simulink model "Detumbling"  (R2023b)
settings: Solver=VariableStepAuto  StartTime=0.0  StopTime=10.0  RelTol=1e-3
values from neighbouring files (symbols this model uses):
  a = 7259    [Group_51.m]
  ARW = (((arw*pi/180)/(sqrt(n_t)))^2)*n_t    [Group_51.m]
  Beta_CMG = acos(dot([1;0;0],uv_pyr))    [Group_51.m]
  delta_0_D = zeros(4,1)    [Group_51.m]
  e = 0.001    [Group_51.m]
  eps_b = 11.5*pi/180    (= 0.200712863979)    [Group_51.m]
  f0 = deg2rad(0)    [Group_51.m]
  g_1_0 = -29404.8    [Group_51.m]
  g_1_1 = -1450.9    [Group_51.m]
  Gain_G = eye(3,3)    [Group_51.m]
  h_1_1 = 4653.5    [Group_51.m]
  h_r = [0.5;0.5;0.5;0.5]    [Group_51.m]
  halfrange = pi/40    (= 0.0785398163397)    [Group_51.m]
  i = deg2rad(97.27276)    [Group_51.m]
  I = diag(I)    [Group_51.m]
  I_inv = I\eye(3,3)    [Group_51.m]
  IC312_D = [phi312_D;theta312_D;psi312_D]    [Group_51.m]
  jb = [0.1; 0.1;0.1]    [Group_51.m]
  k_cmg = -1    [Group_51.m]
  kdx_D = 0.9896    [Group_51.m]
  kdy_D = 0.9734    [Group_51.m]
  kdz_D = 0.9096    [Group_51.m]
  Miss_G = [teta_g_x;teta_g_y;teta_g_z]    [Group_51.m]
  n = sqrt(mu/ a^3)    [Group_51.m]
  n_t = samp_t    (= 1)    [Group_51.m]
  OM = deg2rad(90)    [Group_51.m]
  Re = astroConstants(23)    [Group_51.m]
  RRW = (((rrw*pi/180)/(sqrt(n_t)))^2)*n_t    [Group_51.m]
  samp_t = 1/samp_freq    (= 1)    [Group_51.m]
  w = deg2rad(0)    [Group_51.m]
  w0_D = [wx_D;wy_D;wz_D]    [Group_51.m]
  w_t_D = zeros(3,1)    [Group_51.m]
  we = we/3600    (= 7.29159776389e-06)    [Group_51.m]
undefined symbols (not defined in the file or in its folder): DiscIntNeverNeededParam
libraries: matrix_library x7, vrlib x4, simulink x2, hdlsllib x2, dspswit3 x1
(part 1 of 2)
settings Model: Creator=leo-deo  LastModifiedBy=leo-deo

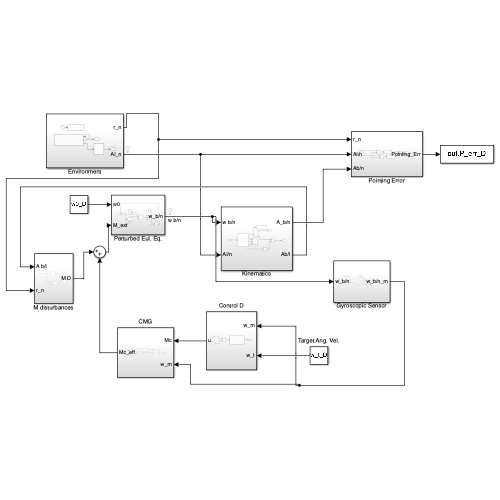
[thumbnail: Simulink's stored preview of the top-level diagram]
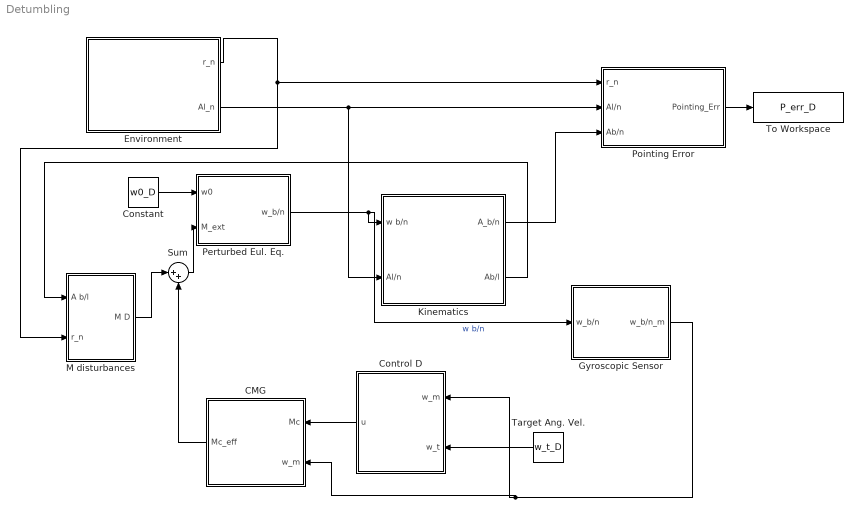
== system Detumbling ==
  CMG : Subsystem
  Constant : Constant  Value=w0_D
  Control D : Subsystem
  Environment : Subsystem
  Gyroscopic Sensor : Subsystem
  Kinematics : Subsystem
  M disturbances : Subsystem
  Perturbed Eul. Eq. : Subsystem
  Pointing Error : Subsystem
  Sum : Sum  Inputs=|++
  Target Ang. Vel. : Constant  Value=w_t_D
  To Workspace : ToWorkspace  VariableName=P_err_D  SampleTime=-1
  wires:
  Constant/1 -> Perturbed Eul. Eq./1(w0)
  Sum/1 -> Perturbed Eul. Eq./2(M_ext)
  CMG/1(Mc_eff) -> Sum/2
  Environment/1(r_n) -> Pointing Error/1(r_n), M disturbances/2(r_n)
  Kinematics/2(Ab/l) -> M disturbances/1(A b/l)
  M disturbances/1(M D) -> Sum/1
  Control D/1(u) -> CMG/1(Mc)
  Environment/2(Al_n) -> Kinematics/2(Al/n), Pointing Error/2(Al/n)
  Gyroscopic Sensor/1(w_b/n_m) -> CMG/2(w_m), Control D/1(w_m)
  Target Ang. Vel./1 -> Control D/2(w_t)
  Perturbed Eul. Eq./1(w_b/n) -> Gyroscopic Sensor/1(w_b/n), Kinematics/1(w b/n)  "w b/n"
  Pointing Error/1(Pointing_Err) -> To Workspace/1
  Kinematics/1(A_b/n) -> Pointing Error/3(Ab/n)

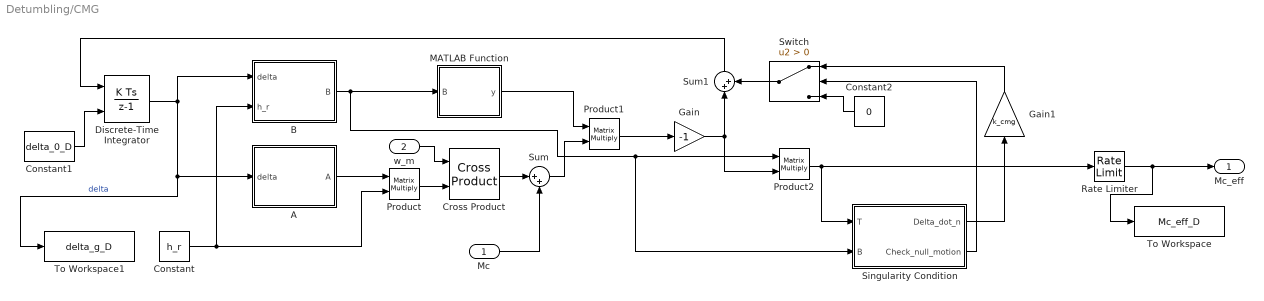
== system Detumbling/CMG ==
  Mc : Inport
  w_m : Inport  Port=2
  A : Subsystem
  B : Subsystem
  Constant : Constant  Value=h_r
  Constant1 : Constant  Value=delta_0_D
  Constant2 : Constant  Value=0
  Cross Product : matrix_library/Cross Product
  Discrete-Time Integrator : DiscreteIntegrator  InitialConditionSource=external  SampleTime=-1  ICPrevOutput=DiscIntNeverNeededParam  ICPrevScaledInput=DiscIntNeverNeededParam
  Gain : Gain  Gain=-1
  Gain1 : Gain  Gain=k_cmg
  MATLAB Function : MATLAB Function  TreatAsAtomicUnit=on
  Product : Product  Multiplication=Matrix(*)
  Product1 : Product  Multiplication=Matrix(*)
  Product2 : Product  Multiplication=Matrix(*)
  Rate Limiter : RateLimiter
  Singularity Condition : Subsystem
  Sum : Sum  Inputs=|++
  Sum1 : Sum  Inputs=|++
  Switch : Switch  Criteria=u2 > Threshold  SaturateOnIntegerOverflow=off  InputSameDT=off
  To Workspace : ToWorkspace  VariableName=Mc_eff_D  SampleTime=-1
  To Workspace1 : ToWorkspace  VariableName=delta_g_D  SampleTime=-1
  Mc_eff : Outport
  wires:
  Rate Limiter/1 -> To Workspace/1, Mc_eff/1
  MATLAB Function/1(y) -> Product1/1
  Discrete-Time Integrator/1 -> B/1(delta), To Workspace1/1, A/1(delta)  "delta"
  w_m/1 -> Cross Product/1
  Cross Product/1 -> Sum/1
  Sum/1 -> Product1/2
  Product1/1 -> Gain/1
  Constant/1 -> B/2(h_r), Product/2
  B/1(B) -> MATLAB Function/1(B), Singularity Condition/2(B), Product2/1
  Product/1 -> Cross Product/2
  A/1(A) -> Product/1
  Gain/1 -> Sum1/1, Product2/2
  Constant1/1 -> Discrete-Time Integrator/2
  Sum1/1 -> Discrete-Time Integrator/1
  Switch/1 -> Sum1/2
  Constant2/1 -> Switch/3
  Singularity Condition/2(Check_null_motion) -> Switch/2
  Singularity Condition/1(Delta_dot_n) -> Gain1/1
  Gain1/1 -> Switch/1
  Mc/1 -> Sum/2
  Product2/1 -> Rate Limiter/1, Singularity Condition/1(T)

== system Detumbling/Control D ==
  w_m : Inport
  w_t : Inport  Port=2
  P : Subsystem
  Subtract : Sum  Inputs=+-
  u : Outport
  wires:
  Subtract/1 -> P/1(Alpha_dot)
  w_t/1 -> Subtract/2
  w_m/1 -> Subtract/1
  P/1(u) -> u/1

== system Detumbling/Environment ==
  A l/n for elliptical orbit : Subsystem
  Clock : Clock
  Kep 2bp : Subsystem
  Terminator : Terminator
  To Workspace : ToWorkspace  VariableName=t_D  SampleTime=-1
  r_n : Outport
  Al_n : Outport  Port=2
  wires:
  Kep 2bp/1(r_n) -> r_n/1
  A l/n for elliptical orbit/2(Al/n) -> Al_n/1
  Clock/1 -> To Workspace/1
  A l/n for elliptical orbit/3(Theta) -> Kep 2bp/1(Theta)
  A l/n for elliptical orbit/1(wl) -> Terminator/1

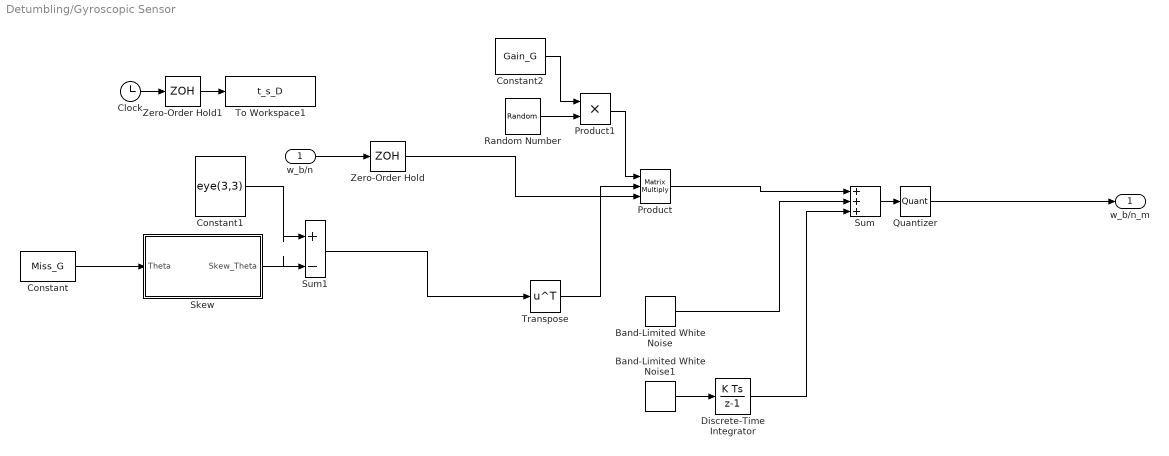
== system Detumbling/Gyroscopic Sensor ==
  w_b/n : Inport
  Band-Limited White Noise : simulink/Sources/Band-Limited White Noise  Cov=[ARW]  Ts=n_t  seed=[23341]
  Band-Limited White Noise1 : simulink/Sources/Band-Limited White Noise  Cov=[RRW]  Ts=n_t  seed=[23341]
  Clock : Clock
  Constant : Constant  Value=Miss_G
  Constant1 : Constant  Value=eye(3,3)
  Constant2 : Constant  Value=Gain_G
  Discrete-Time Integrator : DiscreteIntegrator  SampleTime=-1  ICPrevOutput=DiscIntNeverNeededParam  ICPrevScaledInput=DiscIntNeverNeededParam
  Product : Product  Inputs=3  Multiplication=Matrix(*)
  Product1 : Product
  Quantizer : Quantizer  QuantizationInterval=Gs_res
  Random Number : RandomNumber  Mean=1  Variance=0.0005  SampleTime=n_t
  Skew : Subsystem
  Sum : Sum  Inputs=|+|+||+
  Sum1 : Sum  Inputs=||+||-||
  To Workspace1 : ToWorkspace  VariableName=t_s_D  SampleTime=-1
  Transpose : Math  Operator=transpose
  Zero-Order Hold : ZeroOrderHold  SampleTime=samp_t
  Zero-Order Hold1 : ZeroOrderHold  SampleTime=samp_t
  w_b/n_m : Outport
  wires:
  Band-Limited White Noise1/1 -> Discrete-Time Integrator/1
  Band-Limited White Noise/1 -> Sum/2
  Constant2/1 -> Product1/1
  Random Number/1 -> Product1/2
  Product1/1 -> Product/1
  Product/1 -> Sum/1
  Sum/1 -> Quantizer/1
  w_b/n/1 -> Zero-Order Hold/1
  Sum1/1 -> Transpose/1
  Discrete-Time Integrator/1 -> Sum/3
  Constant1/1 -> Sum1/1
  Skew/1(Skew_Theta) -> Sum1/2
  Constant/1 -> Skew/1(Theta)
  Quantizer/1 -> w_b/n_m/1
  Zero-Order Hold/1 -> Product/3
  Transpose/1 -> Product/2
  Clock/1 -> Zero-Order Hold1/1
  Zero-Order Hold1/1 -> To Workspace1/1

== system Detumbling/Kinematics ==
  w b/n : Inport
  Al/n : Inport  Port=2
  Euler Angles : Subsystem
  Product2 : Product  Multiplication=Matrix(*)
  Subsystem : Subsystem
  To Workspace : ToWorkspace  VariableName=A_bn_D  SampleTime=-1
  Transpose1 : Math  Operator=transpose
  A_b/n : Outport
  Ab/l : Outport  Port=2
  wires:
  w b/n/1 -> Euler Angles/1(w_b)
  Al/n/1 -> Transpose1/1
  Transpose1/1 -> Product2/2
  Product2/1 -> Ab/l/1  "Ab/l"
  Euler Angles/3(Ang_313) -> Subsystem/2(Ang_313)
  Euler Angles/1(A_b/n) -> Product2/1, A_b/n/1, To Workspace/1
  Euler Angles/2(Ang_312) -> Subsystem/1(Ang_312)
  Euler Angles/4(T-F) -> Subsystem/3(T-F)

== system Detumbling/M disturbances ==
  A b/l : Inport
  r_n : Inport  Port=2
  M of B : Subsystem
  M of G G : Subsystem
  Sum : Sum  Inputs=||+||+||
  M D : Outport
  wires:
  Sum/1 -> M D/1
  A b/l/1 -> M of B/1(A b/n), M of G G/1(Ab/l)
  r_n/1 -> M of B/2(r_n)
  M of G G/1(M_G_G) -> Sum/1
  M of B/1(M B) -> Sum/2

== system Detumbling/Perturbed Eul. Eq. ==
  w0 : Inport
  M_ext : Inport  Port=2
  Constant2 : Constant  Value=I
  Constant3 : Constant  Value=I_inv
  Cross Product : matrix_library/Cross Product
  Integrator1 : Integrator  InitialConditionSource=external  AbsoluteTolerance=1e-10
  Product : Product  Multiplication=Matrix(*)
  Product1 : Product  Multiplication=Matrix(*)
  Product2 : Product  Multiplication=Matrix(*)
  Sum : Sum  Inputs=|-+
  To Workspace : ToWorkspace  VariableName=w_b_D  SampleTime=-1
  w_b/n : Outport
  wires:
  Constant2/1 -> Product/1
  Product/1 -> Cross Product/2
  Product2/1 -> Sum/2
  Sum/1 -> Integrator1/1
  Constant3/1 -> Product2/1, Product1/1
  Cross Product/1 -> Product1/2
  Integrator1/1 -> Cross Product/1, Product/2, To Workspace/1, w_b/n/1
  Product1/1 -> Sum/1
  w0/1 -> Integrator1/2
  M_ext/1 -> Product2/2

== system Detumbling/Pointing Error ==
  r_n : Inport
  Al/n : Inport  Port=2
  Ab/n : Inport  Port=3
  Acos : Trigonometry  Operator=acos
  Dot Product : DotProduct  OutDataTypeStr=Inherit: Inherit via internal rule
  Normalize Vector : vrlib/Utilities/Normalize Vector  maxzero=0
  Normalize Vector1 : vrlib/Utilities/Normalize Vector  maxzero=0
  Product : Product  Multiplication=Matrix(*)
  Product1 : Product  Multiplication=Matrix(*)
  Pointing_Err : Outport
  wires:
  Ab/n/1 -> Product1/1
  Al/n/1 -> Product/1
  Normalize Vector/1 -> Dot Product/2
  Product1/1 -> Normalize Vector/1
  Dot Product/1 -> Acos/1
  r_n/1 -> Product/2, Product1/2
  Normalize Vector1/1 -> Dot Product/1
  Product/1 -> Normalize Vector1/1
  Acos/1 -> Pointing_Err/1

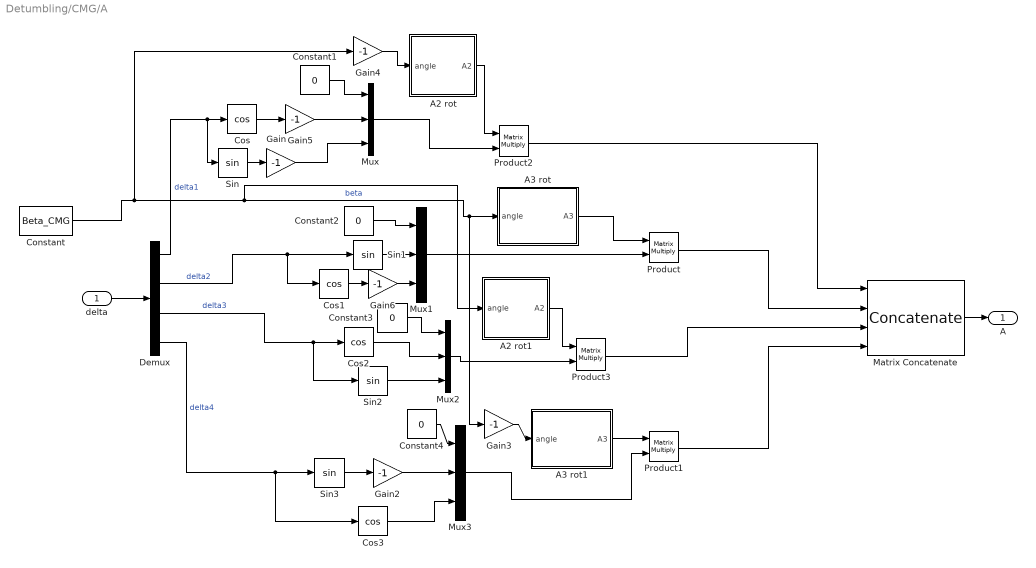
== system Detumbling/CMG/A ==
  delta : Inport
  A2 rot : Subsystem
  A2 rot1 : Subsystem
  A3 rot : Subsystem
  A3 rot1 : Subsystem
  Constant : Constant  Value=Beta_CMG
  Constant{1..4} (4 alike) : Constant  Value=0
  Cos{,1..3} (4 alike) : Trigonometry  Operator=cos
  Demux : Demux
  Gain{,2..6} (6 alike) : Gain  Gain=-1
  Matrix Concatenate : Concatenate  NumInputs=4  Mode=Multidimensional array  ConcatenateDimension=2
  Mux{,1..3} (4 alike) : Mux  Inputs=3
  Product{,1..3} (4 alike) : Product  Multiplication=Matrix(*)
  Sin{,1..3} (4 alike) : Trigonometry
  A : Outport
  wires:
  Constant4/1 -> Mux3/1
  Constant2/1 -> Mux1/1
  Sin3/1 -> Gain2/1
  Sin/1 -> Gain/1
  delta/1 -> Demux/1
  Demux/1 -> Sin/1, Cos/1  "delta1"
  Gain/1 -> Mux/3
  Constant1/1 -> Mux/1
  Constant3/1 -> Mux2/1
  Sin1/1 -> Mux1/2
  Demux/2 -> Cos1/1, Sin1/1  "delta2"
  Cos3/1 -> Mux3/3
  Gain2/1 -> Mux3/2
  Demux/4 -> Cos3/1, Sin3/1  "delta4"
  Mux1/1 -> Product/2
  Constant/1 -> Gain4/1, A2 rot1/1(angle), Gain3/1, A3 rot/1(angle)  "beta"
  A3 rot/1(A3) -> Product/1
  Product/1 -> Matrix Concatenate/2
  Gain3/1 -> A3 rot1/1(angle)
  A3 rot1/1(A3) -> Product1/1
  Mux3/1 -> Product1/2
  Product1/1 -> Matrix Concatenate/4
  A2 rot/1(A2) -> Product2/1
  Mux/1 -> Product2/2
  Gain4/1 -> A2 rot/1(angle)
  Product2/1 -> Matrix Concatenate/1
  Mux2/1 -> Product3/2
  Product3/1 -> Matrix Concatenate/3
  A2 rot1/1(A2) -> Product3/1
  Matrix Concatenate/1 -> A/1
  Gain5/1 -> Mux/2
  Cos/1 -> Gain5/1
  Gain6/1 -> Mux1/3
  Cos1/1 -> Gain6/1
  Sin2/1 -> Mux2/3
  Cos2/1 -> Mux2/2
  Demux/3 -> Sin2/1, Cos2/1  "delta3"

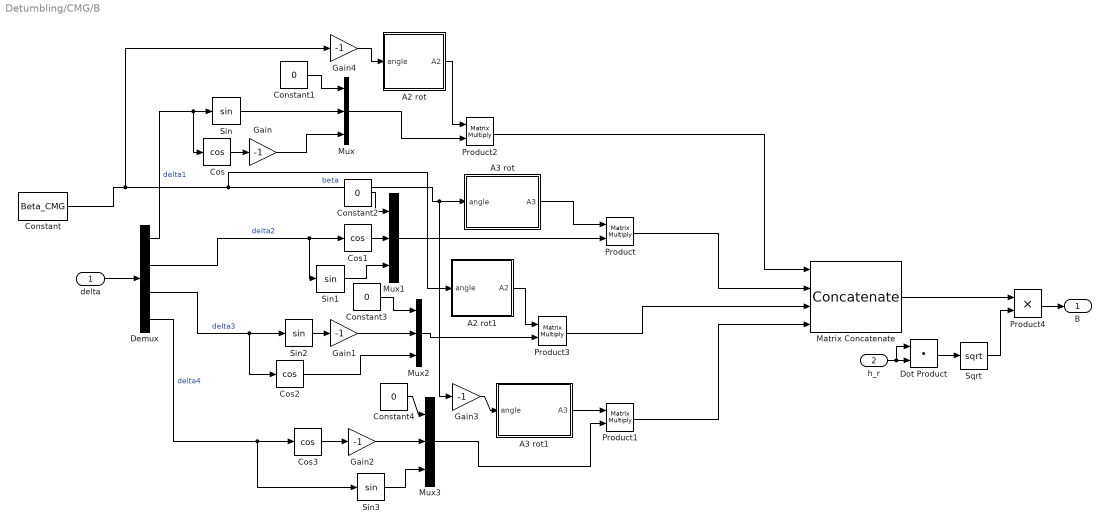
== system Detumbling/CMG/B ==
  delta : Inport
  h_r : Inport  Port=2
  A2 rot : Subsystem
  A2 rot1 : Subsystem
  A3 rot : Subsystem
  A3 rot1 : Subsystem
  Constant : Constant  Value=Beta_CMG
  Constant{1..4} (4 alike) : Constant  Value=0
  Cos{,1..3} (4 alike) : Trigonometry  Operator=cos
  Demux : Demux
  Dot Product : DotProduct  OutDataTypeStr=Inherit: Inherit via internal rule
  Gain{,1..4} (5 alike) : Gain  Gain=-1
  Matrix Concatenate : Concatenate  NumInputs=4  Mode=Multidimensional array  ConcatenateDimension=2
  Mux{,1..3} (4 alike) : Mux  Inputs=3
  Product{,1..3} (4 alike) : Product  Multiplication=Matrix(*)
  Product4 : Product
  Sin{,1..3} (4 alike) : Trigonometry
  Sqrt : Sqrt
  B : Outport
  wires:
  Constant4/1 -> Mux3/1
  Sin1/1 -> Mux1/3
  Constant2/1 -> Mux1/1
  Cos3/1 -> Gain2/1
  Cos/1 -> Gain/1
  delta/1 -> Demux/1
  Demux/1 -> Cos/1, Sin/1  "delta1"
  Gain/1 -> Mux/3
  Gain1/1 -> Mux2/2
  Constant1/1 -> Mux/1
  Constant3/1 -> Mux2/1
  Cos1/1 -> Mux1/2
  Demux/2 -> Cos1/1, Sin1/1  "delta2"
  Sin3/1 -> Mux3/3
  Cos2/1 -> Mux2/3
  Gain2/1 -> Mux3/2
  Sin/1 -> Mux/2
  Demux/4 -> Sin3/1, Cos3/1  "delta4"
  Sin2/1 -> Gain1/1
  Demux/3 -> Cos2/1, Sin2/1  "delta3"
  Mux1/1 -> Product/2
  Constant/1 -> Gain4/1, A2 rot1/1(angle), Gain3/1, A3 rot/1(angle)  "beta"
  A3 rot/1(A3) -> Product/1
  Product/1 -> Matrix Concatenate/2
  Gain3/1 -> A3 rot1/1(angle)
  A3 rot1/1(A3) -> Product1/1
  Mux3/1 -> Product1/2
  Product1/1 -> Matrix Concatenate/4
  A2 rot/1(A2) -> Product2/1
  Mux/1 -> Product2/2
  Gain4/1 -> A2 rot/1(angle)
  Product2/1 -> Matrix Concatenate/1
  Mux2/1 -> Product3/2
  Product3/1 -> Matrix Concatenate/3
  A2 rot1/1(A2) -> Product3/1
  Product4/1 -> B/1
  Matrix Concatenate/1 -> Product4/1
  h_r/1 -> Dot Product/1, Dot Product/2
  Dot Product/1 -> Sqrt/1
  Sqrt/1 -> Product4/2

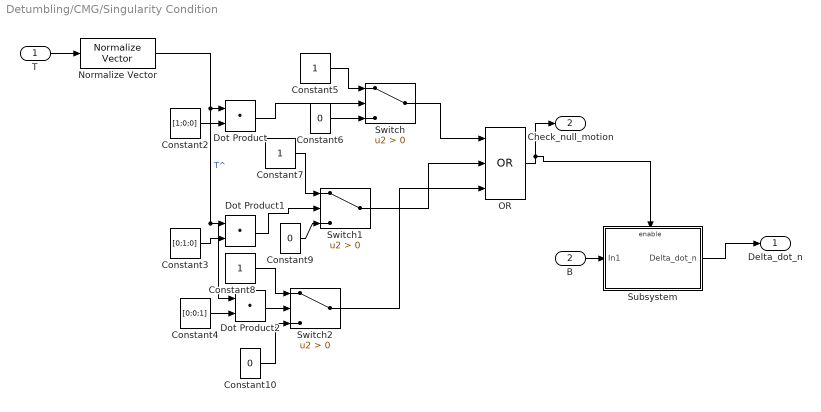
== system Detumbling/CMG/Singularity Condition ==
  T : Inport
  B : Inport  Port=2
  Constant10 : Constant  Value=0
  Constant2 : Constant  Value=[1;0;0]
  Constant3 : Constant  Value=[0;1;0]
  Constant4 : Constant  Value=[0;0;1]
  Constant5 : Constant
  Constant6 : Constant  Value=0
  Constant7 : Constant
  Constant8 : Constant
  Constant9 : Constant  Value=0
  Dot Product : DotProduct  OutDataTypeStr=Inherit: Inherit via internal rule
  Dot Product1 : DotProduct  OutDataTypeStr=Inherit: Inherit via internal rule
  Dot Product2 : DotProduct  OutDataTypeStr=Inherit: Inherit via internal rule
  Normalize Vector : vrlib/Utilities/Normalize Vector  maxzero=0
  OR : Logic  Operator=OR  Inputs=3  IconShape=distinctive  AllPortsSameDT=off  OutDataTypeStr=boolean
  Subsystem : Subsystem
  Switch : Switch  Criteria=u2 > Threshold  SaturateOnIntegerOverflow=off  InputSameDT=off
  Switch1 : Switch  Criteria=u2 > Threshold  SaturateOnIntegerOverflow=off  InputSameDT=off
  Switch2 : Switch  Criteria=u2 > Threshold  SaturateOnIntegerOverflow=off  InputSameDT=off
  Delta_dot_n : Outport
  Check_null_motion : Outport  Port=2
  wires:
  Constant2/1 -> Dot Product/2
  T/1 -> Normalize Vector/1
  Constant3/1 -> Dot Product1/2
  Switch2/1 -> OR/3
  Constant9/1 -> Switch1/3
  Dot Product1/1 -> Switch1/2
  Switch1/1 -> OR/2
  Normalize Vector/1 -> Dot Product2/1, Dot Product1/1, Dot Product/1  "T^"
  Dot Product2/1 -> Switch2/2
  Dot Product/1 -> Switch/2
  Constant8/1 -> Switch2/1
  Switch/1 -> OR/1
  Constant5/1 -> Switch/1
  Constant4/1 -> Dot Product2/2
  Constant6/1 -> Switch/3
  Constant7/1 -> Switch1/1
  Constant10/1 -> Switch2/3
  OR/1 -> Subsystem/Enable, Check_null_motion/1
  Subsystem/1(Delta_dot_n) -> Delta_dot_n/1
  B/1 -> Subsystem/1(In1)

== system Detumbling/Control D/P ==
  Alpha_dot : Inport
  Demux : Demux  Outputs=3
  Gain : Gain  Gain=kdx_D
  Gain1 : Gain  Gain=kdy_D
  Gain2 : Gain  Gain=kdz_D
  Mux : Mux  Inputs=3
  u : Outport
  wires:
  Alpha_dot/1 -> Demux/1
  Demux/1 -> Gain/1
  Demux/2 -> Gain1/1
  Mux/1 -> u/1
  Gain/1 -> Mux/1
  Gain1/1 -> Mux/2
  Gain2/1 -> Mux/3
  Demux/3 -> Gain2/1

== system Detumbling/Environment/A l//n for elliptical orbit ==
  Arg. of perigee : Constant  Value=w
  Constant : Constant  Value=[0;0;1]
  Constant3 : Constant  Value=f0
  Inclination : Constant  Value=i
  Product : Product
  RAAN : Constant  Value=OM
  Subsystem : Subsystem
  Subsystem1 : Subsystem
  Sum : Sum  Inputs=|++
  To Workspace : ToWorkspace  VariableName=Theta_D  SampleTime=-1
  wl : Outport
  Al/n : Outport  Port=2
  Theta : Outport  Port=3
  wires:
  Constant3/1 -> Subsystem/1(True Anomaly0)
  Constant/1 -> Product/2
  RAAN/1 -> Subsystem1/1(OM)
  Inclination/1 -> Subsystem1/2(i)
  Arg. of perigee/1 -> Sum/1
  Sum/1 -> Subsystem1/3(w+f)
  Subsystem/1(theta) -> To Workspace/1, Sum/2, Theta/1  "true anomaly"
  Subsystem/2(teta_dot) -> Product/1
  Subsystem1/1(A313) -> Al/n/1
  Product/1 -> wl/1

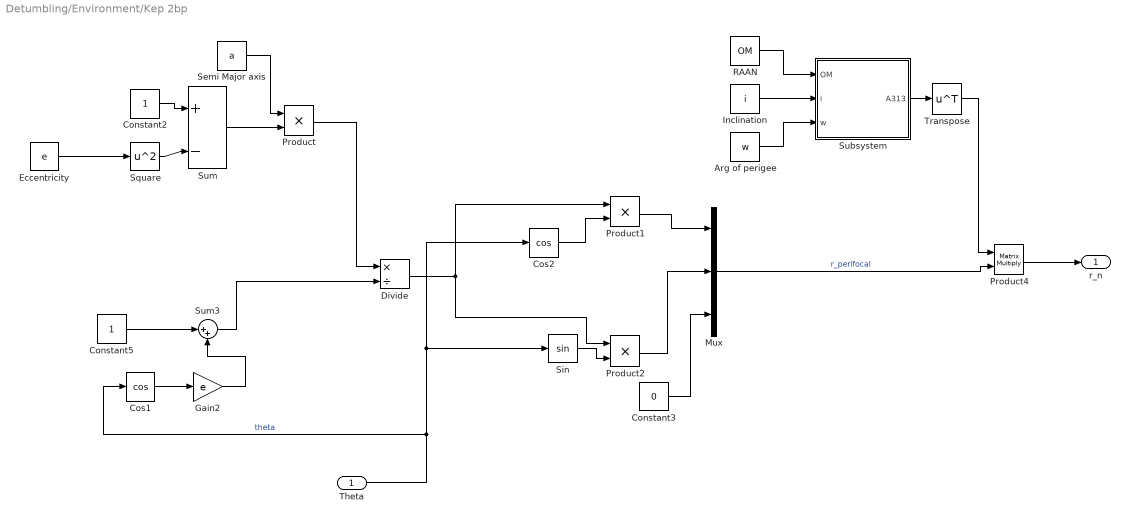
== system Detumbling/Environment/Kep 2bp ==
  Theta : Inport
  Arg of perigee : Constant  Value=w
  Constant2 : Constant
  Constant3 : Constant  Value=0
  Constant5 : Constant
  Cos1 : Trigonometry  Operator=cos
  Cos2 : Trigonometry  Operator=cos
  Divide : Product  Inputs=*/
  Eccentricity : Constant  Value=e
  Gain2 : Gain  Gain=e
  Inclination : Constant  Value=i
  Mux : Mux  Inputs=3
  Product : Product
  Product1 : Product
  Product2 : Product
  Product4 : Product  Multiplication=Matrix(*)
  RAAN : Constant  Value=OM
  Semi Major axis : Constant  Value=a
  Sin : Trigonometry
  Square : Math  Operator=square
  Subsystem : Subsystem
  Sum : Sum  Inputs=|+-
  Sum3 : Sum  Inputs=|++
  Transpose : Math  Operator=transpose
  r_n : Outport
  wires:
  Cos2/1 -> Product1/2
  Eccentricity/1 -> Square/1
  Sum/1 -> Product/2
  RAAN/1 -> Subsystem/1(OM)
  Product1/1 -> Mux/1
  Cos1/1 -> Gain2/1
  Constant2/1 -> Sum/1
  Product/1 -> Divide/1
  Constant5/1 -> Sum3/1
  Sin/1 -> Product2/2
  Theta/1 -> Cos1/1, Sin/1, Cos2/1  "theta"
  Square/1 -> Sum/2
  Gain2/1 -> Sum3/2
  Sum3/1 -> Divide/2
  Product2/1 -> Mux/2
  Semi Major axis/1 -> Product/1
  Divide/1 -> Product2/1, Product1/1
  Subsystem/1(A313) -> Transpose/1
  Arg of perigee/1 -> Subsystem/3(w)
  Product4/1 -> r_n/1
  Inclination/1 -> Subsystem/2(i)
  Constant3/1 -> Mux/3
  Mux/1 -> Product4/2  "r_perifocal"
  Transpose/1 -> Product4/1

== system Detumbling/Gyroscopic Sensor/Skew ==
  Theta : Inport
  Constant1 : Constant  Value=[1;0;0]
  Constant2 : Constant  Value=[0;1;0]
  Constant3 : Constant  Value=[0;0;1]
  Cross Product : matrix_library/Cross Product
  Cross Product1 : matrix_library/Cross Product
  Cross Product2 : matrix_library/Cross Product
  Matrix Concatenate : Concatenate  NumInputs=3  Mode=Multidimensional array  ConcatenateDimension=2
  Skew_Theta : Outport
  wires:
  Cross Product/1 -> Matrix Concatenate/1
  Constant3/1 -> Cross Product2/2
  Constant1/1 -> Cross Product/2
  Cross Product1/1 -> Matrix Concatenate/2
  Matrix Concatenate/1 -> Skew_Theta/1
  Theta/1 -> Cross Product1/1, Cross Product2/1, Cross Product/1
  Cross Product2/1 -> Matrix Concatenate/3
  Constant2/1 -> Cross Product1/2

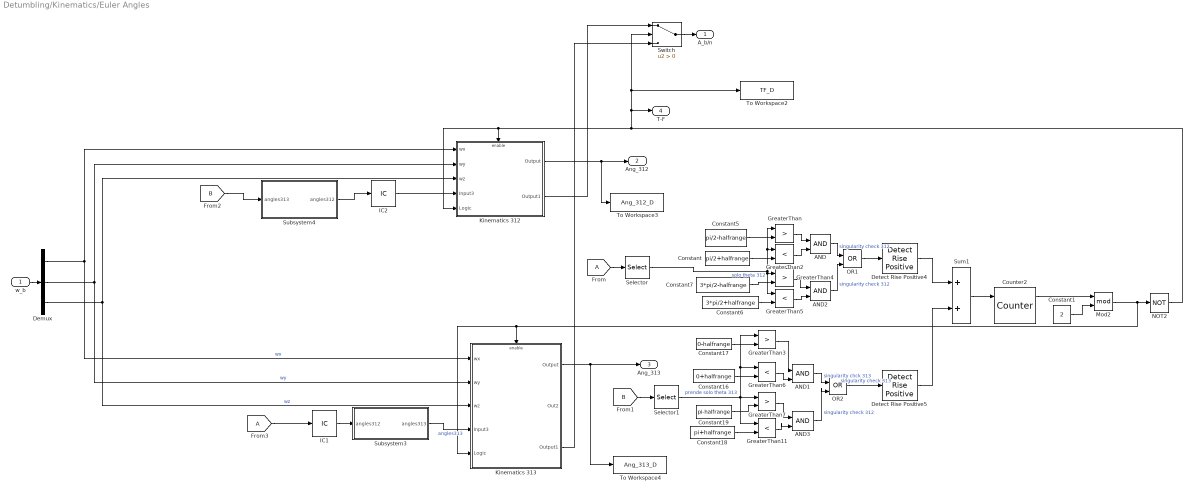
== system Detumbling/Kinematics/Euler Angles ==
  w_b : Inport
  AND{,1..3} (4 alike) : Logic  IconShape=distinctive  AllPortsSameDT=off  OutDataTypeStr=boolean
  Constant : Constant  Value=pi/2+halfrange
  Constant1 : Constant  Value=2
  Constant16 : Constant  Value=0+halfrange
  Constant17 : Constant  Value=0-halfrange
  Constant18 : Constant  Value=pi+halfrange
  Constant19 : Constant  Value=pi-halfrange
  Constant5 : Constant  Value=pi/2-halfrange
  Constant6 : Constant  Value=3*pi/2+halfrange
  Constant7 : Constant  Value=3*pi/2-halfrange
  Counter2 : dspswit3/Counter  Direction=Up  CountEvent=Rising edge  CounterSize=User defined  MaxCount=255  InitialCount=0  Output=Count and Hit  HitValue=32  ResetInput=on  SamplesPerFrame=1  Ts=1  CntDtype=double  HitDtype=Logical
  Demux : Demux  Outputs=3
  Detect Rise Positive4 : hdlsllib/Logic and Bit Operations/Detect Rise Positive  vinit=0  OutDataTypeStr=boolean
  Detect Rise Positive5 : hdlsllib/Logic and Bit Operations/Detect Rise Positive  vinit=0  OutDataTypeStr=boolean
  From : From  TagVisibility=global
  From3 : From  TagVisibility=global
  GreaterThan{,3..4,7} (4 alike) : RelationalOperator  Operator=>  OutDataTypeStr=boolean  RndMeth=Simplest  InputSameDT=off
  GreaterThan{2,5..6,11} (4 alike) : RelationalOperator  Operator=<  OutDataTypeStr=boolean  RndMeth=Simplest  InputSameDT=off
  IC1 : InitialCondition  Value=IC312_D
  IC2 : InitialCondition  Value=IC312_D
  Kinematics 312 : Subsystem
  Kinematics 313 : Subsystem
  Mod2 : Math  Operator=mod
  NOT2 : Logic  Operator=NOT  AllPortsSameDT=off  OutDataTypeStr=boolean
  OR1 : Logic  Operator=OR  IconShape=distinctive  AllPortsSameDT=off  OutDataTypeStr=boolean
  OR2 : Logic  Operator=OR  IconShape=distinctive  AllPortsSameDT=off  OutDataTypeStr=boolean
  Selector : Selector  InputPortWidth=3  IndexOptions=Index vector (dialog)  Indices=2  OutputSizes=1
  Selector1 : Selector  InputPortWidth=3  IndexOptions=Index vector (dialog)  Indices=2  OutputSizes=1
  Subsystem3 : Subsystem
  Subsystem4 : Subsystem
  Sum1 : Sum
  Switch : Switch  Criteria=u2 > Threshold  SaturateOnIntegerOverflow=off  InputSameDT=off
  To Workspace2 : ToWorkspace  VariableName=TF_D  SampleTime=-1
  To Workspace3 : ToWorkspace  VariableName=Ang_312_D  SampleTime=-1
  To Workspace4 : ToWorkspace  VariableName=Ang_313_D  SampleTime=-1
  A_b/n : Outport
  Ang_312 : Outport  Port=2
  Ang_313 : Outport  Port=3
  T-F : Outport  Port=4
  wires:
  Constant5/1 -> GreaterThan/2
  [B] -> Subsystem4/1(angles313)
  Demux/2 -> Kinematics 313/2(wy), Kinematics 312/2(wy)  "wy"
  Sum1/1 -> Counter2/1
  From3/1 -> IC1/1
  OR2/1 -> Detect Rise Positive5/1  "singularity check 313"
  From/1 -> Selector/1
  Selector1/1 -> GreaterThan11/1, GreaterThan3/1, GreaterThan6/1, GreaterThan7/1  "prende solo theta 313"
  Constant/1 -> GreaterThan2/2
  GreaterThan6/1 -> AND1/2
  Constant6/1 -> GreaterThan5/2
  Subsystem4/1(angles312) -> IC2/1
  Counter2/1 -> Mod2/1
  Constant7/1 -> GreaterThan4/2
  IC1/1 -> Subsystem3/1(angles312)
  Constant19/1 -> GreaterThan7/2
  AND/1 -> OR1/1  "singularity check 312"
  Subsystem3/1(angles313) -> Kinematics 313/4(Input3)  "angles313"
  GreaterThan11/1 -> AND3/2
  AND1/1 -> OR2/1  "singularity chck 313"
  GreaterThan4/1 -> AND2/1
  Demux/3 -> Kinematics 313/3(wz), Kinematics 312/3(wz)  "wz"
  Detect Rise Positive5/1 -> Sum1/2
  Constant16/1 -> GreaterThan6/2
  IC2/1 -> Kinematics 312/4(Input3)
  GreaterThan2/1 -> AND/2
  Constant17/1 -> GreaterThan3/2
  Constant1/1 -> Mod2/2
  Selector/1 -> GreaterThan/1, GreaterThan2/1, GreaterThan5/1, GreaterThan4/1  "solo theta 312"
  GreaterThan7/1 -> AND3/1
  NOT2/1 -> T-F/1, Switch/2, To Workspace2/1, Kinematics 312/5(Logic), Kinematics 312/Enable
  OR1/1 -> Detect Rise Positive4/1
  GreaterThan3/1 -> AND1/1
  Constant18/1 -> GreaterThan11/2
  GreaterThan/1 -> AND/1
  Demux/1 -> Kinematics 313/1(wx), Kinematics 312/1(wx)  "wx"
  AND2/1 -> OR1/2  "singularity check 312"
  AND3/1 -> OR2/2  "singularity check 312"
  [B] -> Selector1/1
  Mod2/1 -> Kinematics 313/Enable, Kinematics 313/5(Logic), NOT2/1
  Kinematics 312/2(Output1) -> Switch/1
  GreaterThan5/1 -> AND2/2
  Detect Rise Positive4/1 -> Sum1/1
  w_b/1 -> Demux/1
  Switch/1 -> A_b/n/1
  Kinematics 313/3(Output1) -> Switch/3
  Kinematics 312/1(Output) -> To Workspace3/1, Ang_312/1
  Kinematics 313/1(Output) -> To Workspace4/1, Ang_313/1

== system Detumbling/Kinematics/Subsystem ==
  Ang_312 : Inport
  Ang_313 : Inport  Port=2
  T-F : Inport  Port=3
  Constant : Constant
  Constant1 : Constant  Value=0
  Constant2 : Constant
  Constant3 : Constant  Value=0
  Gain : Gain  Gain=-1
  Subsystem : Subsystem
  Subsystem4 : Subsystem
  Switch : Switch  Criteria=u2 > Threshold  SaturateOnIntegerOverflow=off  InputSameDT=off
  Switch1 : Switch  SaturateOnIntegerOverflow=off  InputSameDT=off
  To Workspace : ToWorkspace  VariableName=Ang_312_into_312_D  SampleTime=-1
  To Workspace1 : ToWorkspace  VariableName=Ang_313_into_312_D  SampleTime=-1
  wires:
  Constant/1 -> Switch/1
  Constant1/1 -> Switch/3
  Ang_312/1 -> Subsystem/1(Ang_312)
  Switch/1 -> Subsystem/Enable
  Subsystem/1(Ang312) -> To Workspace/1
  Ang_313/1 -> Subsystem4/1(angles313)
  Subsystem4/1(angles312) -> To Workspace1/1
  Gain/1 -> Switch1/2
  T-F/1 -> Gain/1, Switch/2
  Constant2/1 -> Switch1/1
  Constant3/1 -> Switch1/3
  Switch1/1 -> Subsystem4/Enable

== system Detumbling/M disturbances/M of B ==
  A b/n : Inport
  r_n : Inport  Port=2
  "B field " : Subsystem
  Cross Product : matrix_library/Cross Product
  Induction current : Constant  Value=jb
  M B : Outport
  wires:
  Cross Product/1 -> M B/1
  A b/n/1 -> "B field "/1(A b/n)
  "B field "/1(b_b) -> Cross Product/2
  Induction current/1 -> Cross Product/1
  r_n/1 -> "B field "/2(r_n)

== system Detumbling/M disturbances/M of G G ==
  Ab/l : Inport
  Constant1 : Constant  Value=I
  Cross Product : matrix_library/Cross Product
  "D.C. of R " : Subsystem
  Gain : Gain  Gain=3
  Mean Angular Speed : Constant  Value=n
  Product1 : Product  Multiplication=Matrix(*)
  Product2 : Product
  Square : Math  Operator=square
  M_G_G : Outport
  wires:
  Mean Angular Speed/1 -> Square/1
  Square/1 -> Gain/1
  Product1/1 -> Cross Product/2
  Ab/l/1 -> "D.C. of R "/1(Ab/l)
  "D.C. of R "/1(c) -> Product1/2, Cross Product/1  "c"
  Gain/1 -> Product2/2  "3*n^2"
  Product2/1 -> M_G_G/1
  Constant1/1 -> Product1/1
  Cross Product/1 -> Product2/1

== system Detumbling/CMG/A/A2 rot ==
  angle : Inport
  Constant5 : Constant  Value=[0 0 0; 0 1 0; 0 0 0]
  Constant6 : Constant  Value=[1 0 0; 0 0 0; 0 0 1]
  Constant7 : Constant  Value=[0 0 1; 0 0 0; -1 0 0]
  Cos4 : Trigonometry  Operator=cos
  Product2 : Product
  Product3 : Product
  Sin4 : Trigonometry
  Sum : Sum  Inputs=|+||+||+
  A2 : Outport
  wires:
  Cos4/1 -> Product2/1
  Product2/1 -> Sum/2
  Constant7/1 -> Product3/2
  Sum/1 -> A2/1
  angle/1 -> Sin4/1, Cos4/1
  Constant6/1 -> Product2/2
  Sin4/1 -> Product3/1
  Product3/1 -> Sum/3
  Constant5/1 -> Sum/1

== system Detumbling/CMG/A/A2 rot1 ==
  angle : Inport
  Constant5 : Constant  Value=[0 0 0; 0 1 0; 0 0 0]
  Constant6 : Constant  Value=[1 0 0; 0 0 0; 0 0 1]
  Constant7 : Constant  Value=[0 0 1; 0 0 0; -1 0 0]
  Cos4 : Trigonometry  Operator=cos
  Product2 : Product
  Product3 : Product
  Sin4 : Trigonometry
  Sum : Sum  Inputs=|+||+||+
  A2 : Outport
  wires:
  Cos4/1 -> Product2/1
  Product2/1 -> Sum/2
  Constant7/1 -> Product3/2
  Sum/1 -> A2/1
  angle/1 -> Sin4/1, Cos4/1
  Constant6/1 -> Product2/2
  Sin4/1 -> Product3/1
  Product3/1 -> Sum/3
  Constant5/1 -> Sum/1

== system Detumbling/CMG/A/A3 rot ==
  angle : Inport
  Constant1 : Constant  Value=[0 0 0; 0 0 0; 0 0 1]
  Constant2 : Constant  Value=[1 0 0; 0 1 0; 0 0 0]
  Constant3 : Constant  Value=[0 1 0; -1 0 0; 0 0 0]
  Cos : Trigonometry  Operator=cos
  Product : Product
  Product1 : Product
  Sin : Trigonometry
  Sum : Sum  Inputs=|+||+||+
  A3 : Outport
  wires:
  Constant2/1 -> Product/2
  Sum/1 -> A3/1
  angle/1 -> Sin/1, Cos/1
  Product/1 -> Sum/2
  Cos/1 -> Product/1
  Sin/1 -> Product1/1
  Constant3/1 -> Product1/2
  Constant1/1 -> Sum/1
  Product1/1 -> Sum/3

== system Detumbling/CMG/A/A3 rot1 ==
  angle : Inport
  Constant1 : Constant  Value=[0 0 0; 0 0 0; 0 0 1]
  Constant2 : Constant  Value=[1 0 0; 0 1 0; 0 0 0]
  Constant3 : Constant  Value=[0 1 0; -1 0 0; 0 0 0]
  Cos : Trigonometry  Operator=cos
  Product : Product
  Product1 : Product
  Sin : Trigonometry
  Sum : Sum  Inputs=|+||+||+
  A3 : Outport
  wires:
  Constant2/1 -> Product/2
  Sum/1 -> A3/1
  angle/1 -> Sin/1, Cos/1
  Product/1 -> Sum/2
  Cos/1 -> Product/1
  Sin/1 -> Product1/1
  Constant3/1 -> Product1/2
  Constant1/1 -> Sum/1
  Product1/1 -> Sum/3

== system Detumbling/CMG/B/A2 rot ==
  angle : Inport
  Constant5 : Constant  Value=[0 0 0; 0 1 0; 0 0 0]
  Constant6 : Constant  Value=[1 0 0; 0 0 0; 0 0 1]
  Constant7 : Constant  Value=[0 0 1; 0 0 0; -1 0 0]
  Cos4 : Trigonometry  Operator=cos
  Product2 : Product
  Product3 : Product
  Sin4 : Trigonometry
  Sum : Sum  Inputs=|+||+||+
  A2 : Outport
  wires:
  Cos4/1 -> Product2/1
  Product2/1 -> Sum/2
  Constant7/1 -> Product3/2
  Sum/1 -> A2/1
  angle/1 -> Sin4/1, Cos4/1
  Constant6/1 -> Product2/2
  Sin4/1 -> Product3/1
  Product3/1 -> Sum/3
  Constant5/1 -> Sum/1

== system Detumbling/CMG/B/A2 rot1 ==
  angle : Inport
  Constant5 : Constant  Value=[0 0 0; 0 1 0; 0 0 0]
  Constant6 : Constant  Value=[1 0 0; 0 0 0; 0 0 1]
  Constant7 : Constant  Value=[0 0 1; 0 0 0; -1 0 0]
  Cos4 : Trigonometry  Operator=cos
  Product2 : Product
  Product3 : Product
  Sin4 : Trigonometry
  Sum : Sum  Inputs=|+||+||+
  A2 : Outport
  wires:
  Cos4/1 -> Product2/1
  Product2/1 -> Sum/2
  Constant7/1 -> Product3/2
  Sum/1 -> A2/1
  angle/1 -> Sin4/1, Cos4/1
  Constant6/1 -> Product2/2
  Sin4/1 -> Product3/1
  Product3/1 -> Sum/3
  Constant5/1 -> Sum/1

== system Detumbling/CMG/B/A3 rot ==
  angle : Inport
  Constant1 : Constant  Value=[0 0 0; 0 0 0; 0 0 1]
  Constant2 : Constant  Value=[1 0 0; 0 1 0; 0 0 0]
  Constant3 : Constant  Value=[0 1 0; -1 0 0; 0 0 0]
  Cos : Trigonometry  Operator=cos
  Product : Product
  Product1 : Product
  Sin : Trigonometry
  Sum : Sum  Inputs=|+||+||+
  A3 : Outport
  wires:
  Constant2/1 -> Product/2
  Sum/1 -> A3/1
  angle/1 -> Sin/1, Cos/1
  Product/1 -> Sum/2
  Cos/1 -> Product/1
  Sin/1 -> Product1/1
  Constant3/1 -> Product1/2
  Constant1/1 -> Sum/1
  Product1/1 -> Sum/3

== system Detumbling/CMG/B/A3 rot1 ==
  angle : Inport
  Constant1 : Constant  Value=[0 0 0; 0 0 0; 0 0 1]
  Constant2 : Constant  Value=[1 0 0; 0 1 0; 0 0 0]
  Constant3 : Constant  Value=[0 1 0; -1 0 0; 0 0 0]
  Cos : Trigonometry  Operator=cos
  Product : Product
  Product1 : Product
  Sin : Trigonometry
  Sum : Sum  Inputs=|+||+||+
  A3 : Outport
  wires:
  Constant2/1 -> Product/2
  Sum/1 -> A3/1
  angle/1 -> Sin/1, Cos/1
  Product/1 -> Sum/2
  Cos/1 -> Product/1
  Sin/1 -> Product1/1
  Constant3/1 -> Product1/2
  Constant1/1 -> Sum/1
  Product1/1 -> Sum/3

== system Detumbling/CMG/Singularity Condition/Subsystem ==
  In1 : Inport
  Enable : EnablePort
  Constant : Constant  Value=[0;0;0]
  MATLAB Function : MATLAB Function  TreatAsAtomicUnit=on
  Product : Product  Multiplication=Matrix(*)
  Delta_dot_n : Outport
  wires:
  MATLAB Function/1(y) -> Product/1
  Product/1 -> Delta_dot_n/1
  In1/1 -> MATLAB Function/1(B)
  Constant/1 -> Product/2

== system Detumbling/Environment/A l//n for elliptical orbit/Subsystem ==
  True Anomaly0 : Inport
  Constant : Constant
  Constant1 : Constant
  Constant5 : Constant  Value=3/2
  Cos1 : Trigonometry  Operator=cos
  Divide1 : Product  Inputs=*/
  Earth rotation rate : Gain  Gain=we
  Eccentricity : Constant  Value=e
  Gain : Gain  Gain=e
  Integrator : Integrator  InitialConditionSource=external
  Power : Math  Operator=pow
  Square : Math  Operator=square
  Square1 : Math  Operator=square
  Sum2 : Sum  Inputs=|++
  Sum3 : Sum  Inputs=|+-
  theta : Outport
  teta_dot : Outport  Port=2
  wires:
  Constant/1 -> Sum2/1
  Eccentricity/1 -> Square/1
  Sum3/1 -> Power/1
  Divide1/1 -> teta_dot/1, Integrator/1
  Cos1/1 -> Gain/1
  Sum2/1 -> Square1/1
  True Anomaly0/1 -> Integrator/2
  Power/1 -> Divide1/2
  Constant1/1 -> Sum3/1
  Square1/1 -> Earth rotation rate/1
  Constant5/1 -> Power/2
  Integrator/1 -> theta/1, Cos1/1  "theta"
  Earth rotation rate/1 -> Divide1/1
  Gain/1 -> Sum2/2
  Square/1 -> Sum3/2

== system Detumbling/Environment/A l//n for elliptical orbit/Subsystem1 ==
  OM : Inport
  i : Inport  Port=2
  w+f : Inport  Port=3
  2 A1 rot : Subsystem
  2 A3 rot : Subsystem
  2 A3 rot2 : Subsystem
  Product : Product  Inputs=3  Multiplication=Matrix(*)
  A313 : Outport
  wires:
  2 A3 rot/1(A23) -> Product/3
  OM/1 -> 2 A3 rot/1(ang)
  Product/1 -> A313/1
  2 A1 rot/1(A21) -> Product/2
  2 A3 rot2/1(A233) -> Product/1
  w+f/1 -> 2 A3 rot2/1(ang)
  i/1 -> 2 A1 rot/1(ang)

== system Detumbling/Environment/Kep 2bp/Subsystem ==
  OM : Inport
  i : Inport  Port=2
  w : Inport  Port=3
  2 A1 rot : Subsystem
  2 A3 rot : Subsystem
  2 A3 rot2 : Subsystem
  Product : Product  Inputs=3  Multiplication=Matrix(*)
  A313 : Outport
  wires:
  2 A3 rot/1(A23) -> Product/3
  OM/1 -> 2 A3 rot/1(angolo)
  Product/1 -> A313/1
  2 A1 rot/1(A21) -> Product/2
  2 A3 rot2/1(A233) -> Product/1
  w/1 -> 2 A3 rot2/1(angolo)
  i/1 -> 2 A1 rot/1(theta2)

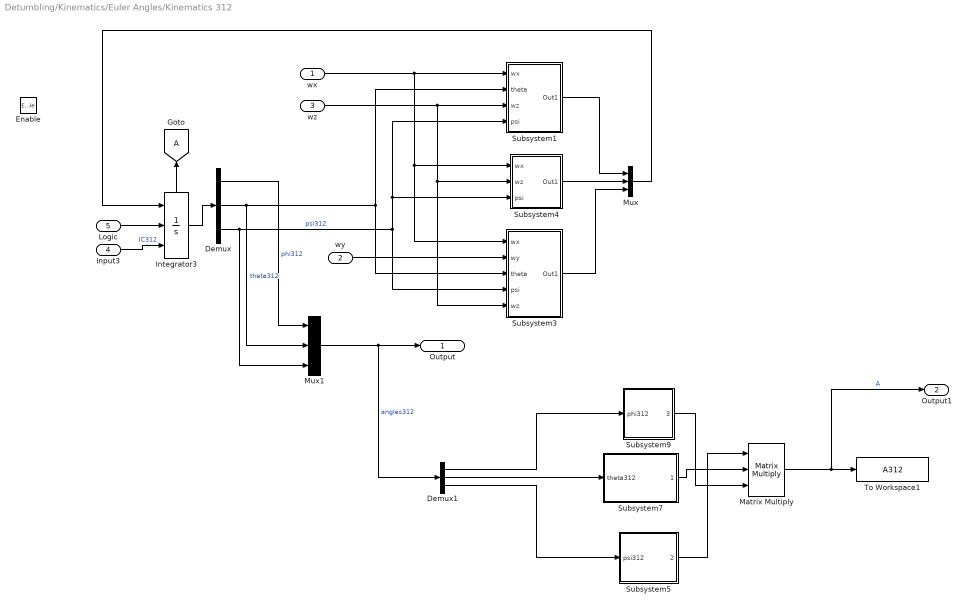
== system Detumbling/Kinematics/Euler Angles/Kinematics 312 ==
  wx : Inport
  wy : Inport  Port=2
  wz : Inport  Port=3
  Input3 : Inport  Port=4
  Logic : Inport  Port=5
  Enable : EnablePort  StatesWhenEnabling=reset
  Demux : Demux  Outputs=3
  Demux1 : Demux  Outputs=3
  Goto : Goto  TagVisibility=global
  Integrator3 : Integrator  ExternalReset=rising  InitialConditionSource=external  ShowStatePort=on
  Matrix Multiply : Product  Inputs=3  Multiplication=Matrix(*)
  Mux : Mux  Inputs=3
  Mux1 : Mux  Inputs=3
  Subsystem1 : Subsystem
  Subsystem3 : Subsystem
  Subsystem4 : Subsystem
  Subsystem5 : Subsystem
  Subsystem7 : Subsystem
  Subsystem9 : Subsystem
  To Workspace1 : ToWorkspace  VariableName=A312  SampleTime=-1
  Output : Outport
  Output1 : Outport  Port=2
  wires:
  Integrator3/1 -> Demux/1
  Integrator3/State -> Goto/1
  Demux/1 -> Mux1/1  "phi312"
  Demux/2 -> Mux1/2, Subsystem1/2(theta), Subsystem3/3(theta)  "theta312"
  Demux/3 -> Mux1/3, Subsystem1/4(psi), Subsystem4/3(psi), Subsystem3/4(psi)  "psi312"
  wx/1 -> Subsystem3/1(wx), Subsystem4/1(wx), Subsystem1/1(wx)
  wz/1 -> Subsystem3/5(wz), Subsystem4/2(wz), Subsystem1/3(wz)
  wy/1 -> Subsystem3/2(wy)
  Subsystem1/1(Out1) -> Mux/1
  Subsystem4/1(Out1) -> Mux/2
  Subsystem3/1(Out1) -> Mux/3
  Mux/1 -> Integrator3/1
  Mux1/1 -> Demux1/1, Output/1  "angles312"
  Input3/1 -> Integrator3/3  "IC312"
  Logic/1 -> Integrator3/2
  Demux1/3 -> Subsystem5/1(psi312)
  Subsystem9/1(3) -> Matrix Multiply/3
  Subsystem5/1(2) -> Matrix Multiply/1
  Demux1/2 -> Subsystem7/1(theta312)
  Demux1/1 -> Subsystem9/1(phi312)
  Subsystem7/1(1) -> Matrix Multiply/2
  Matrix Multiply/1 -> Output1/1, To Workspace1/1  "A"

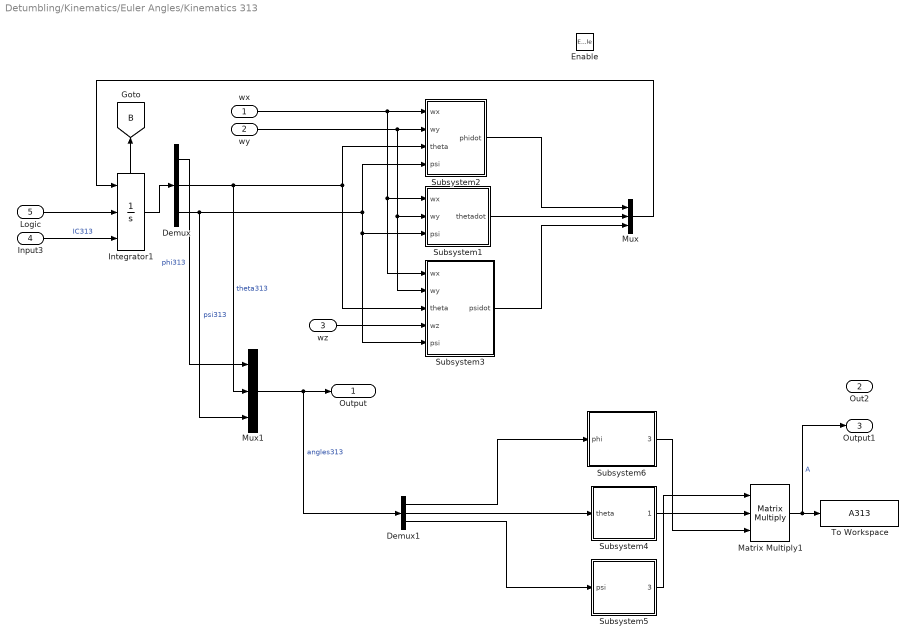
== system Detumbling/Kinematics/Euler Angles/Kinematics 313 ==
  wx : Inport
  wy : Inport  Port=2
  wz : Inport  Port=3
  Input3 : Inport  Port=4
  Logic : Inport  Port=5
  Enable : EnablePort  StatesWhenEnabling=reset
  Demux : Demux  Outputs=3
  Demux1 : Demux  Outputs=3
  Integrator1 : Integrator  ExternalReset=rising  InitialConditionSource=external  ShowStatePort=on
  Matrix Multiply1 : Product  Inputs=3  Multiplication=Matrix(*)
  Mux : Mux  Inputs=3
  Mux1 : Mux  Inputs=3
  Subsystem1 : Subsystem
  Subsystem2 : Subsystem
  Subsystem3 : Subsystem
  Subsystem4 : Subsystem
  Subsystem5 : Subsystem
  Subsystem6 : Subsystem
  To Workspace : ToWorkspace  VariableName=A313  SampleTime=-1
  Output : Outport
  Out2 : Outport  Port=2
  Output1 : Outport  Port=3
  tag scope: B=global
  wires:
  Integrator1/State -> [B]
  Integrator1/1 -> Demux/1
  Subsystem3/1(psidot) -> Mux/3
  Subsystem2/1(phidot) -> Mux/1
  Demux/1 -> Mux1/1  "phi313"
  Subsystem1/1(thetadot) -> Mux/2
  Mux/1 -> Integrator1/1
  Demux/2 -> Subsystem3/3(theta), Subsystem2/3(theta), Mux1/2  "theta313"
  Demux/3 -> Mux1/3, Subsystem1/3(psi), Subsystem3/5(psi), Subsystem2/4(psi)  "psi313"
  wx/1 -> Subsystem1/1(wx), Subsystem3/1(wx), Subsystem2/1(wx)
  wy/1 -> Subsystem3/2(wy), Subsystem1/2(wy), Subsystem2/2(wy)
  wz/1 -> Subsystem3/4(wz)
  Mux1/1 -> Demux1/1, Output/1  "angles313"
  Input3/1 -> Integrator1/3  "IC313"
  Logic/1 -> Integrator1/2
  Demux1/2 -> Subsystem4/1(theta)
  Subsystem5/1(3) -> Matrix Multiply1/1
  Subsystem4/1(1) -> Matrix Multiply1/2
  Demux1/3 -> Subsystem5/1(psi)
  Demux1/1 -> Subsystem6/1(phi)
  Subsystem6/1(3) -> Matrix Multiply1/3
  Matrix Multiply1/1 -> Output1/1, To Workspace/1  "A"

== system Detumbling/Kinematics/Euler Angles/Subsystem3 ==
  angles312 : Inport
  Subsystem10 : Subsystem
  Subsystem12 : Subsystem
  Subsystem4 : Subsystem
  Subsystem6 : Subsystem
  angles313 : Outport
  wires:
  Subsystem12/1(Out1) -> Subsystem4/1(matrix313)  "matrix313"
  angles312/1 -> Subsystem6/1(In1)
  Subsystem10/1(angles313) -> Subsystem12/1(angles313)  "angles313"
  Subsystem6/1(Out1) -> Subsystem10/1(In1)
  Subsystem4/1(angles313) -> angles313/1  "angles313"

== system Detumbling/Kinematics/Euler Angles/Subsystem4 ==
  angles313 : Inport
  Subsystem1 : Subsystem
  Subsystem12 : Subsystem
  angles312 : Outport
  wires:
  Subsystem12/1(Out1) -> Subsystem1/1(matrix313)  "matrix313"
  Subsystem1/1(angles312) -> angles312/1  "angles312"
  angles313/1 -> Subsystem12/1(angles313)

== system Detumbling/Kinematics/Subsystem/Subsystem ==
  Ang_312 : Inport
  Enable : EnablePort
  Ang312 : Outport
  wires:
  Ang_312/1 -> Ang312/1

== system Detumbling/Kinematics/Subsystem/Subsystem4 ==
  angles313 : Inport
  Enable : EnablePort
  Subsystem1 : Subsystem
  Subsystem12 : Subsystem
  angles312 : Outport
  wires:
  Subsystem12/1(Out1) -> Subsystem1/1(matrix313)  "matrix313"
  Subsystem1/1(angles312) -> angles312/1  "angles312"
  angles313/1 -> Subsystem12/1(angles313)

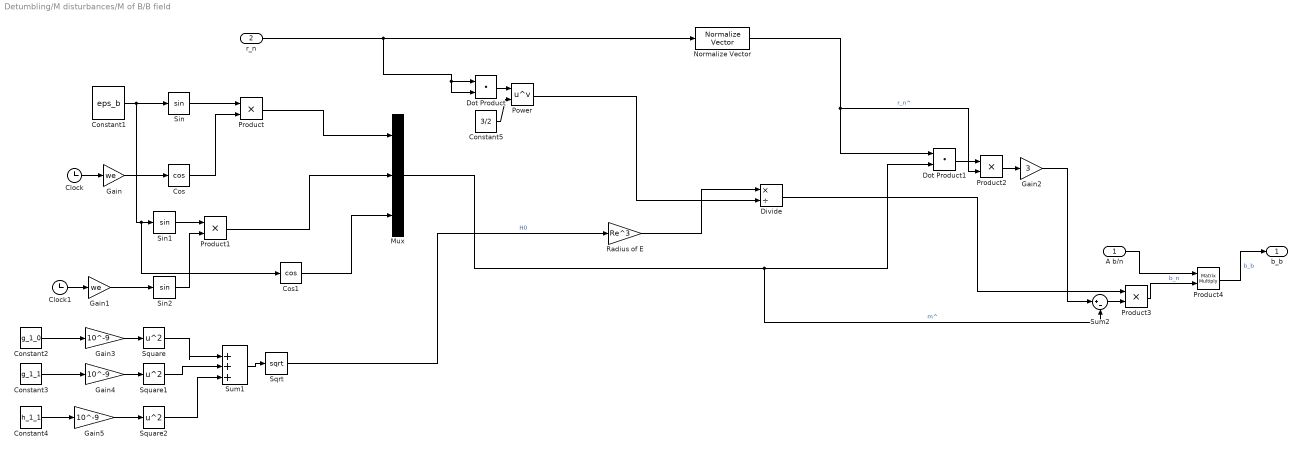
== system Detumbling/M disturbances/M of B/B field  ==
  A b/n : Inport
  r_n : Inport  Port=2
  Clock : Clock
  Clock1 : Clock
  Constant1 : Constant  Value=eps_b
  Constant2 : Constant  Value=g_1_0
  Constant3 : Constant  Value=g_1_1
  Constant4 : Constant  Value=h_1_1
  Constant5 : Constant  Value=3/2
  Cos : Trigonometry  Operator=cos
  Cos1 : Trigonometry  Operator=cos
  Divide : Product  Inputs=*/
  Dot Product : DotProduct  OutDataTypeStr=Inherit: Inherit via internal rule
  Dot Product1 : DotProduct  OutDataTypeStr=Inherit: Inherit via internal rule
  Gain : Gain  Gain=we
  Gain1 : Gain  Gain=we
  Gain2 : Gain  Gain=3
  Gain3 : Gain  Gain=10^-9
  Gain4 : Gain  Gain=10^-9
  Gain5 : Gain  Gain=10^-9
  Mux : Mux  Inputs=3
  Normalize Vector : vrlib/Utilities/Normalize Vector  maxzero=0
  Power : Math  Operator=pow
  Product{,1..3} (4 alike) : Product
  Product4 : Product  Multiplication=Matrix(*)
  Radius of E : Gain  Gain=Re^3
  Sin : Trigonometry
  Sin1 : Trigonometry
  Sin2 : Trigonometry
  Sqrt : Sqrt
  Square : Math  Operator=square
  Square1 : Math  Operator=square
  Square2 : Math  Operator=square
  Sum1 : Sum  Inputs=|+++
  Sum2 : Sum  Inputs=|+-
  b_b : Outport
  wires:
  A b/n/1 -> Product4/1
  Product2/1 -> Gain2/1
  Constant5/1 -> Power/2
  Radius of E/1 -> Divide/1
  Normalize Vector/1 -> Product2/2, Dot Product1/1  "r_n^"
  Gain/1 -> Cos/1
  Sum2/1 -> Product3/2
  Sin1/1 -> Product1/1
  Product1/1 -> Mux/2
  Sqrt/1 -> Radius of E/1  "H0"
  Clock/1 -> Gain/1
  Gain1/1 -> Sin2/1
  Sin2/1 -> Product1/2
  Sin/1 -> Product/1
  Product4/1 -> b_b/1  "b_b"
  Clock1/1 -> Gain1/1
  Cos/1 -> Product/2
  Square2/1 -> Sum1/3
  Constant1/1 -> Cos1/1, Sin1/1, Sin/1
  Cos1/1 -> Mux/3
  Dot Product/1 -> Power/1
  Product3/1 -> Product4/2  "b_n"
  Divide/1 -> Product3/1
  Product/1 -> Mux/1
  Power/1 -> Divide/2
  Sum1/1 -> Sqrt/1
  Dot Product1/1 -> Product2/1
  r_n/1 -> Normalize Vector/1, Dot Product/2, Dot Product/1
  Square1/1 -> Sum1/2
  Square/1 -> Sum1/1
  Mux/1 -> Sum2/2, Dot Product1/2  "m^"
  Gain2/1 -> Sum2/1
  Constant2/1 -> Gain3/1
  Gain3/1 -> Square/1
  Gain4/1 -> Square1/1
  Constant3/1 -> Gain4/1
  Constant4/1 -> Gain5/1
  Gain5/1 -> Square2/1

== system Detumbling/M disturbances/M of G G/D.C. of R  ==
  Ab/l : Inport
  Product : Product  Multiplication=Matrix(*)
  Yaw Axis : Constant  Value=[1; 0; 0]
  c : Outport
  wires:
  Product/1 -> c/1  "c"
  Ab/l/1 -> Product/1
  Yaw Axis/1 -> Product/2

== system Detumbling/Environment/A l//n for elliptical orbit/Subsystem1/2 A1 rot ==
  ang : Inport
  Constant1 : Constant  Value=[1 0 0; 0 0 0; 0 0 0]
  Constant2 : Constant  Value=[0 0 0; 0 1 0; 0 0 1]
  Constant3 : Constant  Value=[0 0 0; 0 0 1; 0 -1 0]
  Cos : Trigonometry  Operator=cos
  Product : Product
  Product1 : Product
  Sin : Trigonometry
  Sum : Sum  Inputs=|+||+||+
  A21 : Outport
  wires:
  ang/1 -> Sin/1, Cos/1
  Constant3/1 -> Product1/2
  Product1/1 -> Sum/3
  Product/1 -> Sum/2
  Constant1/1 -> Sum/1
  Sin/1 -> Product1/1
  Constant2/1 -> Product/2
  Cos/1 -> Product/1
  Sum/1 -> A21/1

== system Detumbling/Environment/A l//n for elliptical orbit/Subsystem1/2 A3 rot ==
  ang : Inport
  Constant1 : Constant  Value=[0 0 0; 0 0 0; 0 0 1]
  Constant2 : Constant  Value=[1 0 0; 0 1 0; 0 0 0]
  Constant3 : Constant  Value=[0 1 0; -1 0 0; 0 0 0]
  Cos : Trigonometry  Operator=cos
  Product : Product
  Product1 : Product
  Sin : Trigonometry
  Sum : Sum  Inputs=|+||+||+
  A23 : Outport
  wires:
  Constant2/1 -> Product/2
  Sum/1 -> A23/1
  ang/1 -> Sin/1, Cos/1
  Product/1 -> Sum/2
  Cos/1 -> Product/1
  Sin/1 -> Product1/1
  Constant3/1 -> Product1/2
  Constant1/1 -> Sum/1
  Product1/1 -> Sum/3

== system Detumbling/Environment/A l//n for elliptical orbit/Subsystem1/2 A3 rot2 ==
  ang : Inport
  Constant1 : Constant  Value=[0 0 0; 0 0 0; 0 0 1]
  Constant2 : Constant  Value=[1 0 0; 0 1 0; 0 0 0]
  Constant3 : Constant  Value=[0 1 0; -1 0 0; 0 0 0]
  Cos : Trigonometry  Operator=cos
  Product : Product
  Product1 : Product
  Sin : Trigonometry
  Sum : Sum  Inputs=|+||+||+
  A233 : Outport
  wires:
  Constant2/1 -> Product/2
  Sum/1 -> A233/1
  ang/1 -> Sin/1, Cos/1
  Product/1 -> Sum/2
  Cos/1 -> Product/1
  Sin/1 -> Product1/1
  Constant3/1 -> Product1/2
  Constant1/1 -> Sum/1
  Product1/1 -> Sum/3

== system Detumbling/Environment/Kep 2bp/Subsystem/2 A1 rot ==
  theta2 : Inport
  Constant1 : Constant  Value=[1 0 0; 0 0 0; 0 0 0]
  Constant2 : Constant  Value=[0 0 0; 0 1 0; 0 0 1]
  Constant3 : Constant  Value=[0 0 0; 0 0 1; 0 -1 0]
  Cos : Trigonometry  Operator=cos
  Product : Product
  Product1 : Product
  Sin : Trigonometry
  Sum : Sum  Inputs=|+||+||+
  A21 : Outport
  wires:
  theta2/1 -> Sin/1, Cos/1
  Constant3/1 -> Product1/2
  Product1/1 -> Sum/3
  Product/1 -> Sum/2
  Constant1/1 -> Sum/1
  Sin/1 -> Product1/1
  Constant2/1 -> Product/2
  Cos/1 -> Product/1
  Sum/1 -> A21/1

== system Detumbling/Environment/Kep 2bp/Subsystem/2 A3 rot ==
  angolo : Inport
  Constant1 : Constant  Value=[0 0 0; 0 0 0; 0 0 1]
  Constant2 : Constant  Value=[1 0 0; 0 1 0; 0 0 0]
  Constant3 : Constant  Value=[0 1 0; -1 0 0; 0 0 0]
  Cos : Trigonometry  Operator=cos
  Product : Product
  Product1 : Product
  Sin : Trigonometry
  Sum : Sum  Inputs=|+||+||+
  A23 : Outport
  wires:
  Constant2/1 -> Product/2
  Sum/1 -> A23/1
  angolo/1 -> Sin/1, Cos/1
  Product/1 -> Sum/2
  Cos/1 -> Product/1
  Sin/1 -> Product1/1
  Constant3/1 -> Product1/2
  Constant1/1 -> Sum/1
  Product1/1 -> Sum/3

== system Detumbling/Environment/Kep 2bp/Subsystem/2 A3 rot2 ==
  angolo : Inport
  Constant1 : Constant  Value=[0 0 0; 0 0 0; 0 0 1]
  Constant2 : Constant  Value=[1 0 0; 0 1 0; 0 0 0]
  Constant3 : Constant  Value=[0 1 0; -1 0 0; 0 0 0]
  Cos : Trigonometry  Operator=cos
  Product : Product
  Product1 : Product
  Sin : Trigonometry
  Sum : Sum  Inputs=|+||+||+
  A233 : Outport
  wires:
  Constant2/1 -> Product/2
  Sum/1 -> A233/1
  angolo/1 -> Sin/1, Cos/1
  Product/1 -> Sum/2
  Cos/1 -> Product/1
  Sin/1 -> Product1/1
  Constant3/1 -> Product1/2
  Constant1/1 -> Sum/1
  Product1/1 -> Sum/3

== system Detumbling/Kinematics/Euler Angles/Kinematics 312/Subsystem1 ==
  wx : Inport
  theta : Inport  Port=2
  wz : Inport  Port=3
  psi : Inport  Port=4
  Cos : Trigonometry  Operator=cos
  Cos1 : Trigonometry  Operator=cos
  Divide : Product  Inputs=*/
  Product : Product
  Product1 : Product
  Sin : Trigonometry
  Sum : Sum  Inputs=|+-
  Out1 : Outport
  wires:
  psi/1 -> Cos/1, Sin/1
  theta/1 -> Cos1/1
  Product1/1 -> Sum/2
  Sum/1 -> Divide/1
  Product/1 -> Sum/1
  Sin/1 -> Product1/1
  Cos1/1 -> Divide/2
  Cos/1 -> Product/2
  wx/1 -> Product1/2
  wz/1 -> Product/1
  Divide/1 -> Out1/1  "phidot"

== system Detumbling/Kinematics/Euler Angles/Kinematics 312/Subsystem3 ==
  wx : Inport
  wy : Inport  Port=2
  theta : Inport  Port=3
  psi : Inport  Port=4
  wz : Inport  Port=5
  Cos : Trigonometry  Operator=cos
  Cos1 : Trigonometry  Operator=cos
  Divide : Product  Inputs=*/
  Product : Product
  Product1 : Product
  Product2 : Product
  Sin : Trigonometry
  Sin1 : Trigonometry
  Subtract : Sum  Inputs=+-
  Subtract1 : Sum  Inputs=+-
  Out1 : Outport
  wires:
  psi/1 -> Cos/1, Sin/1
  Subtract/1 -> Product2/1
  Sin1/1 -> Divide/1
  Product2/1 -> Subtract1/2
  Sin/1 -> Product1/1
  Cos/1 -> Product/2
  Cos1/1 -> Divide/2
  Subtract1/1 -> Out1/1  "psidot"
  wz/1 -> Product/1
  theta/1 -> Sin1/1, Cos1/1
  Product1/1 -> Subtract/2
  Divide/1 -> Product2/2
  Product/1 -> Subtract/1
  wy/1 -> Subtract1/1
  wx/1 -> Product1/2

== system Detumbling/Kinematics/Euler Angles/Kinematics 312/Subsystem4 ==
  wx : Inport
  wz : Inport  Port=2
  psi : Inport  Port=3
  Cos : Trigonometry  Operator=cos
  Product : Product
  Product1 : Product
  Sin : Trigonometry
  Sum : Sum  Inputs=|++
  Out1 : Outport
  wires:
  Sum/1 -> Out1/1  "thetadot"
  Sin/1 -> Product1/1
  psi/1 -> Sin/1, Cos/1
  Product/1 -> Sum/1
  Product1/1 -> Sum/2
  wx/1 -> Product/1
  Cos/1 -> Product/2
  wz/1 -> Product1/2

== system Detumbling/Kinematics/Euler Angles/Kinematics 312/Subsystem5 ==
  psi312 : Inport
  Constant1 : Constant  Value=[0 0 0; 0 1 0; 0 0 0]
  Constant2 : Constant  Value=[0 0 -1; 0 0 0; 1 0 0]
  Constant3 : Constant  Value=[1 0 0; 0 0 0; 0 0 1]
  Cos : Trigonometry  Operator=cos
  Product : Product
  Product1 : Product
  Sin : Trigonometry
  Sum : Sum  Inputs=|+++
  2 : Outport
  wires:
  Sum/1 -> 2/1  "A2psi"
  psi312/1 -> Cos/1, Sin/1  "psi"
  Constant1/1 -> Sum/1
  Product/1 -> Sum/2
  Constant2/1 -> Product/2
  Sin/1 -> Product/1
  Cos/1 -> Product1/1
  Constant3/1 -> Product1/2
  Product1/1 -> Sum/3

== system Detumbling/Kinematics/Euler Angles/Kinematics 312/Subsystem7 ==
  theta312 : Inport
  Constant1 : Constant  Value=[1 0 0; 0 0 0; 0 0 0]
  Constant2 : Constant  Value=[0 0 0; 0 0 1; 0 -1 0]
  Constant3 : Constant  Value=[0 0 0; 0 1 0; 0 0 1]
  Cos : Trigonometry  Operator=cos
  Product : Product
  Product1 : Product
  Sin : Trigonometry
  Sum : Sum  Inputs=|+++
  1 : Outport
  wires:
  theta312/1 -> Cos/1, Sin/1
  Sum/1 -> 1/1  "A1theta"
  Constant1/1 -> Sum/1
  Sin/1 -> Product/1
  Constant2/1 -> Product/2
  Product/1 -> Sum/2
  Cos/1 -> Product1/1
  Constant3/1 -> Product1/2
  Product1/1 -> Sum/3

== system Detumbling/Kinematics/Euler Angles/Kinematics 312/Subsystem9 ==
  phi312 : Inport
  Constant1 : Constant  Value=[0 0 0; 0 0 0; 0 0 1]
  Constant2 : Constant  Value=[0 1 0; -1 0 0; 0 0 0]
  Constant3 : Constant  Value=[1 0 0; 0 1 0; 0 0 0]
  Cos : Trigonometry  Operator=cos
  Product : Product
  Product1 : Product
  Sin : Trigonometry
  Sum : Sum  Inputs=|+++
  3 : Outport
  wires:
  phi312/1 -> Cos/1, Sin/1
  Constant1/1 -> Sum/1
  Sum/1 -> 3/1  "A3phi"
  Sin/1 -> Product/1
  Constant2/1 -> Product/2
  Product/1 -> Sum/2
  Cos/1 -> Product1/1
  Constant3/1 -> Product1/2
  Product1/1 -> Sum/3

== system Detumbling/Kinematics/Euler Angles/Kinematics 313/Subsystem1 ==
  wx : Inport
  wy : Inport  Port=2
  psi : Inport  Port=3
  Cos : Trigonometry  Operator=cos
  Product : Product
  Product1 : Product
  Sin : Trigonometry
  Subtract : Sum  Inputs=-+
  thetadot : Outport
  wires:
  Product/1 -> Subtract/1
  Product1/1 -> Subtract/2
  psi/1 -> Sin/1, Cos/1
  wy/1 -> Product/1
  wx/1 -> Product1/2
  Cos/1 -> Product1/1
  Subtract/1 -> thetadot/1  "thetadot"
  Sin/1 -> Product/2

== system Detumbling/Kinematics/Euler Angles/Kinematics 313/Subsystem2 ==
  wx : Inport
  wy : Inport  Port=2
  theta : Inport  Port=3
  psi : Inport  Port=4
  Cos : Trigonometry  Operator=cos
  Cos1 : Trigonometry
  Divide : Product  Inputs=*/
  Product : Product
  Product1 : Product
  Sin : Trigonometry
  Sum : Sum  Inputs=|++
  phidot : Outport
  wires:
  psi/1 -> Cos/1, Sin/1
  Cos/1 -> Product/1
  Sum/1 -> Divide/1
  Cos1/1 -> Divide/2
  Product/1 -> Sum/2
  Product1/1 -> Sum/1
  Sin/1 -> Product1/1
  wx/1 -> Product1/2
  wy/1 -> Product/2
  Divide/1 -> phidot/1  "phidot"
  theta/1 -> Cos1/1

== system Detumbling/Kinematics/Euler Angles/Kinematics 313/Subsystem3 ==
  wx : Inport
  wy : Inport  Port=2
  theta : Inport  Port=3
  wz : Inport  Port=4
  psi : Inport  Port=5
  Cos : Trigonometry  Operator=cos
  Cos1 : Trigonometry
  Cos2 : Trigonometry  Operator=cos
  Cos3 : Trigonometry
  Divide : Product  Inputs=*/
  Product : Product
  Product1 : Product
  Product2 : Product
  Sum : Sum  Inputs=|++
  Sum1 : Sum  Inputs=+-
  psidot : Outport
  wires:
  theta/1 -> Cos3/1, Cos2/1
  Product2/1 -> Sum1/2
  Cos/1 -> Product1/1
  Product/1 -> Sum/1
  Cos2/1 -> Divide/1
  psi/1 -> Cos/1, Cos1/1
  Cos3/1 -> Divide/2
  Divide/1 -> Product2/2
  Sum/1 -> Product2/1
  wy/1 -> Product1/2
  Product1/1 -> Sum/2
  Sum1/1 -> psidot/1  "psidot"
  wz/1 -> Sum1/1
  Cos1/1 -> Product/2
  wx/1 -> Product/1

== system Detumbling/Kinematics/Euler Angles/Kinematics 313/Subsystem4 ==
  theta : Inport
  Constant1 : Constant  Value=[1 0 0; 0 0 0; 0 0 0]
  Constant2 : Constant  Value=[0 0 0; 0 0 1; 0 -1 0]
  Constant3 : Constant  Value=[0 0 0; 0 1 0; 0 0 1]
  Cos : Trigonometry  Operator=cos
  Product : Product
  Product1 : Product
  Sin : Trigonometry
  Sum : Sum  Inputs=|+++
  1 : Outport
  wires:
  theta/1 -> Cos/1, Sin/1
  Sum/1 -> 1/1  "A1theta"
  Constant1/1 -> Sum/1
  Sin/1 -> Product/1
  Constant2/1 -> Product/2
  Product/1 -> Sum/2
  Cos/1 -> Product1/1
  Constant3/1 -> Product1/2
  Product1/1 -> Sum/3

== system Detumbling/Kinematics/Euler Angles/Kinematics 313/Subsystem5 ==
  psi : Inport
  Constant1 : Constant  Value=[0 0 0; 0 0 0; 0 0 1]
  Constant2 : Constant  Value=[0 1 0; -1 0 0; 0 0 0]
  Constant3 : Constant  Value=[1 0 0; 0 1 0; 0 0 0]
  Cos : Trigonometry  Operator=cos
  Product : Product
  Product1 : Product
  Sin : Trigonometry
  Sum : Sum  Inputs=|+++
  3 : Outport
  wires:
  Sum/1 -> 3/1  "A3psi"
  psi/1 -> Sin/1, Cos/1  "psi"
  Product1/1 -> Sum/3
  Constant3/1 -> Product1/2
  Sin/1 -> Product/1
  Constant2/1 -> Product/2
  Cos/1 -> Product1/1
  Product/1 -> Sum/2
  Constant1/1 -> Sum/1

== system Detumbling/Kinematics/Euler Angles/Kinematics 313/Subsystem6 ==
  phi : Inport
  Constant1 : Constant  Value=[0 0 0; 0 0 0; 0 0 1]
  Constant2 : Constant  Value=[0 1 0; -1 0 0; 0 0 0]
  Constant3 : Constant  Value=[1 0 0; 0 1 0; 0 0 0]
  Cos : Trigonometry  Operator=cos
  Product : Product
  Product1 : Product
  Sin : Trigonometry
  Sum : Sum  Inputs=|+++
  3 : Outport
  wires:
  phi/1 -> Cos/1, Sin/1
  Constant1/1 -> Sum/1
  Sum/1 -> 3/1  "A3phi"
  Sin/1 -> Product/1
  Constant2/1 -> Product/2
  Product/1 -> Sum/2
  Cos/1 -> Product1/1
  Constant3/1 -> Product1/2
  Product1/1 -> Sum/3
